simulink library "libStabilityAugmentedSystemModel"  (R2020b)
settings: Solver=VariableStepAuto  StartTime=0.0  StopTime=10.0  RelTol=1e-3
undefined symbols (not defined in the file): scheduleData
settings Model: Creator=caatay  LastModifiedBy=caatay

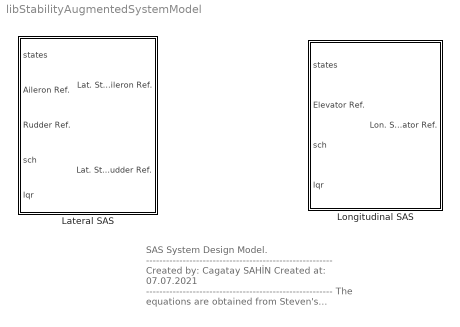
== system libStabilityAugmentedSystemModel ==
  note: SAS System Design Model.
      | --------------------------------------------------------
      | Created by: Cagatay SAHİN
      | Created at: 07.07.2021
      | --------------------------------------------------------
      | The equations are obtained from
      | Steven's textbook.
      | The reference book can be found in
      | "references folder".
      | --------------------------------------------------------
      | for question:
      | cagataysahin44@gmail.com
  Lateral SAS : Subsystem  mask(Flight Control System - Gain Schedule Model -  Lateral Stability Augmented System){scheduleData=scheduleData}
      mask prompts: scheduleData "Schedule Gain Data"
      mask help: Aircraft's lateral stabilization model with using state, sensor information.
      mask Help:
      | This block is used for stabilize aircraft on lateral position with using some informations
      | --------------------------------------------------------------------------------------------------------------------------------------------------
      | Input of the function:
      | 	states: State Information.
      | 	Ref_{i}: Reference Commands.
      | 	Sch: Scheduled Data.
      | 	K_{lqr}: LQR Gain Parameters
      | Output of the function:
      | 	ail: Aileron Deflection (deg)
      | 	rud: Rudder Deflection (deg)
      | --------------------------------------------------------------------------------------------------------------------------------------------------
      | All equations can be found in Steven's text book. Reference can be found in "literature" subfolder.
      | for question: "cagataysahin44@gmail.com"
      mask DialogControl Container2 Prompt: Parameters
      mask Display:
      | port_label('input',1,'states','texmode','on');
      | port_label('input',2,'Ref_{ail}','texmode','on');
      | port_label('input',3,'Ref_{rud}','texmode','on');
      | port_label('input',4,'sch','texmode','on');
      | port_label('input',5,'K_{lqr}','texmode','on');
      | 
      | port_label('output',1,'\delta_{ail_{ref}}','texmode','on');
      | port_label('output',2,'\delta_{rud_{ref}}','texmode','on');
  Longitudinal SAS : Subsystem  mask(Flight Control System - Gain Schedule Model -  Long. Stability Augmented System){scheduleData=scheduleData}
      mask prompts: scheduleData "Schedule Gain Data"
      mask help: Aircraft's longitudinal stabilization model with using state, sensor information.
      mask Help:
      | This block is used for stabilize aircraft on longitudinal position with using some informations
      | --------------------------------------------------------------------------------------------------------------------------------------------------
      | Input of the function:
      | 	states: State Information.
      | 	Ref_{i}: Reference Commands.
      | 	Sch: Scheduled Data.
      | 	K_{lqr}: LQR Gain Parameters
      | Output of the function:
      | 	ele: Elevator Deflection (deg)
      | --------------------------------------------------------------------------------------------------------------------------------------------------
      | All equations can be found in Steven's text book. Reference can be found in "literature" subfolder.
      | for question: "cagataysahin44@gmail.com"
      mask DialogControl Container2 Prompt: Parameters
      mask Display:
      | port_label('input',1,'states','texmode','on');
      | port_label('input',2,'Ref_{ele}','texmode','on');
      | port_label('input',3,'sch','texmode','on');
      | port_label('input',4,'K_{lqr}','texmode','on');
      | 
      | port_label('output',1,'\delta_{ele_{ref}}','texmode','on');

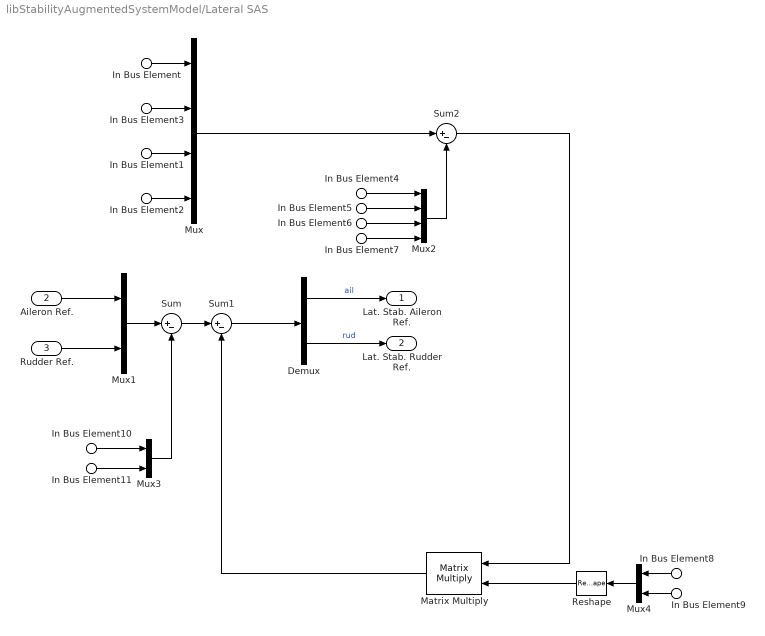
== system libStabilityAugmentedSystemModel/Lateral SAS ==
  In Bus Element : Inport  PortName=states  Element=beta
  In Bus Element1 : Inport  PortName=states  Element=p
  In Bus Element2 : Inport  PortName=states  Element=r
  In Bus Element3 : Inport  PortName=states  Element=phi
  Aileron Ref. : Inport  Port=2
  Rudder Ref. : Inport  Port=3
  In Bus Element4 : Inport  Port=4  PortName=sch  Element=beta
  In Bus Element5 : Inport  Port=4  PortName=sch  Element=phi
  In Bus Element6 : Inport  Port=4  PortName=sch  Element=p
  In Bus Element7 : Inport  Port=4  PortName=sch  Element=r
  In Bus Element10 : Inport  Port=4  PortName=sch  Element=ail
  In Bus Element11 : Inport  Port=4  PortName=sch  Element=rud
  In Bus Element8 : Inport  Port=5  PortName=lqr  Element=lat_ail
  In Bus Element9 : Inport  Port=5  PortName=lqr  Element=lat_rud
  Demux : Demux  Outputs=2
  Matrix Multiply : Product  Multiplication=Matrix(*)
  Mux : Mux
  Mux1 : Mux  Inputs=2
  Mux2 : Mux
  Mux3 : Mux  Inputs=2
  Mux4 : Mux  Inputs=2
  Reshape : Reshape  OutputDimensionality=Customize  OutputDimensions=[4 2]
  Sum : Sum  Inputs=|+-
  Sum1 : Sum  Inputs=|+-
  Sum2 : Sum  Inputs=|+-
  Lat. Stab. Aileron Ref. : Outport  VectorParamsAs1DForOutWhenUnconnected=off
  Lat. Stab. Rudder Ref. : Outport  Port=2  VectorParamsAs1DForOutWhenUnconnected=off
  wires:
  In Bus Element3/1 -> Mux/2
  In Bus Element6/1 -> Mux2/3
  Mux1/1 -> Sum/1
  Demux/1 -> Lat. Stab. Aileron Ref./1  "ail"
  Demux/2 -> Lat. Stab. Rudder Ref./1  "rud"
  Aileron Ref./1 -> Mux1/1
  Sum1/1 -> Demux/1
  In Bus Element7/1 -> Mux2/4
  In Bus Element5/1 -> Mux2/2
  In Bus Element4/1 -> Mux2/1
  Matrix Multiply/1 -> Sum1/2
  In Bus Element11/1 -> Mux3/2
  Mux3/1 -> Sum/2
  Rudder Ref./1 -> Mux1/2
  Sum/1 -> Sum1/1
  Mux2/1 -> Sum2/2
  Mux/1 -> Sum2/1
  In Bus Element2/1 -> Mux/4
  In Bus Element8/1 -> Mux4/1
  In Bus Element9/1 -> Mux4/2
  Sum2/1 -> Matrix Multiply/1
  In Bus Element/1 -> Mux/1
  In Bus Element1/1 -> Mux/3
  Reshape/1 -> Matrix Multiply/2
  Mux4/1 -> Reshape/1
  In Bus Element10/1 -> Mux3/1

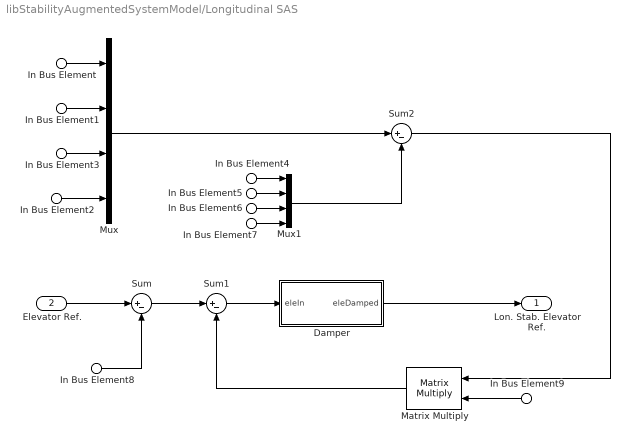
== system libStabilityAugmentedSystemModel/Longitudinal SAS ==
  In Bus Element : Inport  PortName=states  Element=tas
  In Bus Element1 : Inport  PortName=states  Element=alpha
  In Bus Element2 : Inport  PortName=states  Element=q
  In Bus Element3 : Inport  PortName=states  Element=theta
  Elevator Ref. : Inport  Port=2
  In Bus Element4 : Inport  Port=3  PortName=sch  Element=tas
  In Bus Element5 : Inport  Port=3  PortName=sch  Element=alpha
  In Bus Element6 : Inport  Port=3  PortName=sch  Element=theta
  In Bus Element7 : Inport  Port=3  PortName=sch  Element=q
  In Bus Element8 : Inport  Port=3  PortName=sch  Element=ele
  In Bus Element9 : Inport  Port=4  PortName=lqr  Element=lon_ele
  Damper : Subsystem
  Matrix Multiply : Product  Multiplication=Matrix(*)
  Mux : Mux
  Mux1 : Mux
  Sum : Sum  Inputs=|+-
  Sum1 : Sum  Inputs=|+-
  Sum2 : Sum  Inputs=|+-
  Lon. Stab. Elevator Ref. : Outport  VectorParamsAs1DForOutWhenUnconnected=off
  wires:
  Damper/1(eleDamped) -> Lon. Stab. Elevator Ref./1
  In Bus Element3/1 -> Mux/3
  Sum1/1 -> Damper/1(eleIn)
  Elevator Ref./1 -> Sum/1
  Mux/1 -> Sum2/1
  Mux1/1 -> Sum2/2
  In Bus Element1/1 -> Mux/2
  In Bus Element6/1 -> Mux1/3
  In Bus Element2/1 -> Mux/4
  In Bus Element7/1 -> Mux1/4
  In Bus Element8/1 -> Sum/2
  In Bus Element/1 -> Mux/1
  Sum/1 -> Sum1/1
  Matrix Multiply/1 -> Sum1/2
  In Bus Element5/1 -> Mux1/2
  In Bus Element4/1 -> Mux1/1
  In Bus Element9/1 -> Matrix Multiply/2
  Sum2/1 -> Matrix Multiply/1

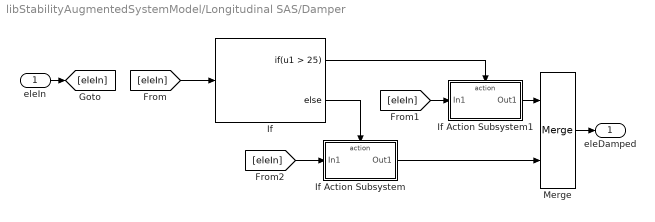
== system libStabilityAugmentedSystemModel/Longitudinal SAS/Damper ==
  eleIn : Inport
  If : If  IfExpression=u1 > 25
  If Action Subsystem : Subsystem  TreatAsAtomicUnit=on
  If Action Subsystem1 : Subsystem  TreatAsAtomicUnit=on
  Merge : Merge
  eleDamped : Outport
  wires:
  eleIn/1 -> [eleIn]
  [eleIn] -> If/1
  If/2 -> If Action Subsystem/Action
  If/1 -> If Action Subsystem1/Action
  [eleIn] -> If Action Subsystem1/1(In1)
  [eleIn] -> If Action Subsystem/1(In1)
  If Action Subsystem1/1(Out1) -> Merge/1
  If Action Subsystem/1(Out1) -> Merge/2
  Merge/1 -> eleDamped/1

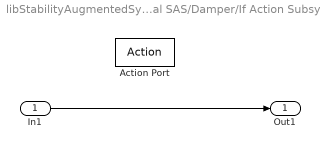
== system libStabilityAugmentedSystemModel/Longitudinal SAS/Damper/If Action Subsystem ==
  In1 : Inport
  Action Port : ActionPort
  Out1 : Outport
  wires:
  In1/1 -> Out1/1

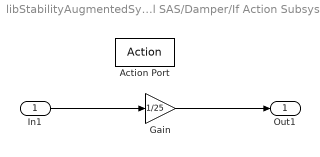
== system libStabilityAugmentedSystemModel/Longitudinal SAS/Damper/If Action Subsystem1 ==
  In1 : Inport
  Action Port : ActionPort
  Gain : Gain  Gain=1/25
  Out1 : Outport
  wires:
  In1/1 -> Gain/1
  Gain/1 -> Out1/1
